simulink model "s462"  (Simulink 5.1)
settings: Solver=ode45  StartTime=0.0  StopTime=200.0  RelTol=1e-3
libraries: simulink x1
settings Model: LastModifiedBy=Administrator  BooleanDataType=on  ProdHWDeviceType=Microprocessor

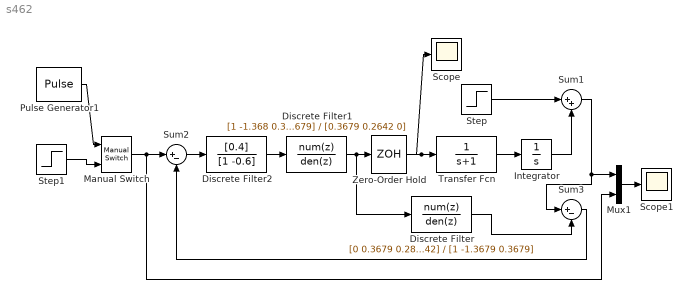
== system s462 ==
  Discrete Filter : DiscreteFilter  Numerator=[0 0.3679 0.2842]  Denominator=[1 -1.3679 0.3679]
  Discrete Filter1 : DiscreteFilter  Numerator=[1 -1.368 0.3679]  Denominator=[0.3679 0.2642 0]
  Discrete Filter2 : DiscreteFilter  Numerator=[0.4]  Denominator=[1 -0.6]
  Integrator : Integrator
  Manual Switch : simulink/Signal Routing/Manual Switch  sw=0  action=0
  Mux1 : Mux  Inputs=2
  Pulse Generator1 : DiscretePulseGenerator  PulseType=Time based  Period=60  PulseWidth=50
  Scope : Scope
      settings: SaveName=ScopeData3
  Scope1 : Scope
  Step : Step  Time=45  After=0.05  SampleTime=0
  Step1 : Step  Time=0  SampleTime=0
  Sum1 : Sum  Inputs=|++  SaturateOnIntegerOverflow=on
  Sum2 : Sum  Inputs=|+-  SaturateOnIntegerOverflow=on
  Sum3 : Sum  Inputs=|+-  SaturateOnIntegerOverflow=on
  Transfer Fcn : TransferFcn  Denominator=[1 1]
  Zero-Order Hold : ZeroOrderHold
  wires:
  Mux1/1 -> Scope1/1
  Discrete Filter1/1 -> Zero-Order Hold/1, Discrete Filter/1
  Sum1/1 -> Mux1/1, Sum3/1
  Sum3/1 -> Sum2/2
  Zero-Order Hold/1 -> Transfer Fcn/1, Scope/1
  Transfer Fcn/1 -> Integrator/1
  Sum2/1 -> Discrete Filter2/1
  Discrete Filter2/1 -> Discrete Filter1/1
  Step/1 -> Sum1/1
  Pulse Generator1/1 -> Manual Switch/1
  Manual Switch/1 -> Sum2/1, Mux1/2
  Step1/1 -> Manual Switch/2
  Discrete Filter/1 -> Sum3/2
  Integrator/1 -> Sum1/2
